simulink model "HW4_Q1_2014a"  (R2022a)
settings: Solver=ode45  StartTime=0.0  StopTime=2000  FixedStep=2  RelTol=1e-3  EnableMultiTasking=on
values from neighbouring files (symbols this model uses):
  proper_Ts = 2    [input_signal.mat]    (also in main.m; prbs_signal.mat; stepResp.mat)
libraries: simulink x1
settings Model: Creator=Sudchai Boonto  LastModifiedBy=Eshmith
settings SolverCC: AlgebraicLoopSolver=TrustRegion
settings DataIOCC: LimitDataPoints=on  SaveFormat=Array  SignalLoggingSaveFormat=ModelDataLogs  ReturnWorkspaceOutputs=off
settings OptimizationCC: ExpressionDepthLimit=2147483647  LifeSpan=inf
settings DebuggingCC: UnderspecifiedInitializationDetection=Classic  MergeDetectMultiDrivingBlocksExec=none  SolverPrmCheckMsg=warning  FcnCallInpInsideContextMsg=warning  UnconnectedInputMsg=warning  UnconnectedOutputMsg=warning  UnconnectedLineMsg=warning  StateNameClashWarn=warning  SFUnexpectedBacktrackingDiag=warning  SFNoUnconditionalDefaultTransitionDiag=warning  SFExecutionAtInitializationDiag=none  SFMachineParentedDataDiag=warning  ArithmeticOperatorsInVariantConditions=warning
settings HardwareCC: ProdBitPerPointer=32  ProdBitPerSizeT=32  ProdBitPerPtrDiffT=32  ProdLargestAtomicFloat=None  ProdIntDivRoundTo=Undefined  ProdEndianess=Unspecified  ProdWordSize=32  ProdHWDeviceType=32-bit Generic
settings ModelReferenceCC: PropagateSignalLabelsOutOfModel=off
settings SFSimCC: SimUseLocalCustomCode=off  CustomCodeUndefinedFunction=UseInterfaceOnly
settings RTWCC: RTWUseLocalCustomCode=off
settings CodeAppCC: StateflowObjectComments=on
settings GRTTargetCC: TargetLangStandard=C89/C90 (ANSI)  CombineOutputUpdateFcns=off  GRTInterface=on
settings ConfigComp: CovMetricSettings=dw  CovSaveCumulativeToWorkspaceVar=on  CovSaveSingleToWorkspaceVar=on  CovExternalEMLEnable=off

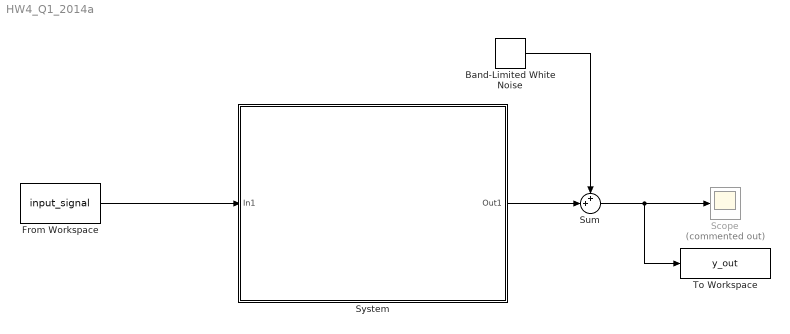
== system HW4_Q1_2014a ==
  Band-Limited White Noise : simulink/Sources/Band-Limited White Noise  Cov=[0.01]  Ts=2  seed=[23341]
  From Workspace : FromWorkspace  VariableName=input_signal  SampleTime=2
  Scope : Scope  Commented=on
  Sum : Sum  Inputs=++|
  System : Subsystem  mask(Rotary Dryer){}
      mask help: This is a rotary dryer for sugar beets. The input to the process is the amount of fuel supplied m_dot and the output is the amount of dry matter phi_DM.
      mask Display: image(imread('dryer.jpg'))
  To Workspace : ToWorkspace  VariableName=y_out  SaveFormat=Timeseries  SampleTime=proper_Ts
  wires:
  System/1(Out1) -> Sum/2
  Band-Limited White Noise/1 -> Sum/1
  From Workspace/1 -> System/1(In1)
  Sum/1 -> To Workspace/1, Scope/1

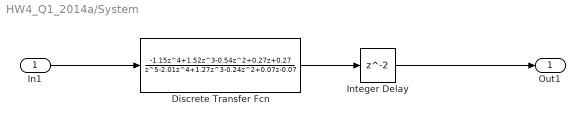
== system HW4_Q1_2014a/System ==
  In1 : Inport
  Discrete Transfer Fcn : DiscreteTransferFcn  Numerator=[-1.15 1.52 -0.54 0.27 0.27]  Denominator="[1  -2.01 1.27 -0.24 0.07 -0.07]"  SampleTime=2
  Integer Delay : Delay
  Out1 : Outport
  wires:
  In1/1 -> Discrete Transfer Fcn/1
  Discrete Transfer Fcn/1 -> Integer Delay/1
  Integer Delay/1 -> Out1/1
